simulink model "AK109_LSQ_simpFric"  (R2025a)
settings: Solver=FixedStepAuto  StartTime=0.0  StopTime=10.0  FixedStep=0.00025  RelTol=1e-3
values from neighbouring files (symbols this model uses):
  b = 1.49    [LSQ_motor_model.m]
  J = 1.59    [LSQ_motor_model.m]
  Kd = Tests(5, index)    [LSQ_motor_model.m]
  Kp = Tests(4, index)    [LSQ_motor_model.m]
  qStepSize = Tests(1, index)    [LSQ_motor_model.m]
  StepTime = 5    [LSQ_motor_model.m]
  wStart = Tests(2, index)    [LSQ_motor_model.m]
  wStepSize = Tests(3, index)    [LSQ_motor_model.m]
undefined symbols (not defined in the file or in its folder): X, Y, Z
libraries: sm_lib x7, nesl_utility x5, fl_lib x4, BalekaSSCs_lib x1
settings Model: Creator=Blue Fifth  LastModifiedBy=Gavin
settings RTWCC: GPUComputeCapability=3.5
settings ExplorerConfigSet: SimMechanicsOpenEditorOnUpdate=off

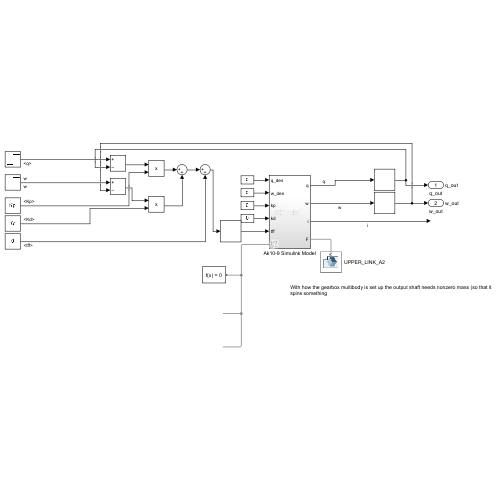
[thumbnail: Simulink's stored preview of the top-level diagram]
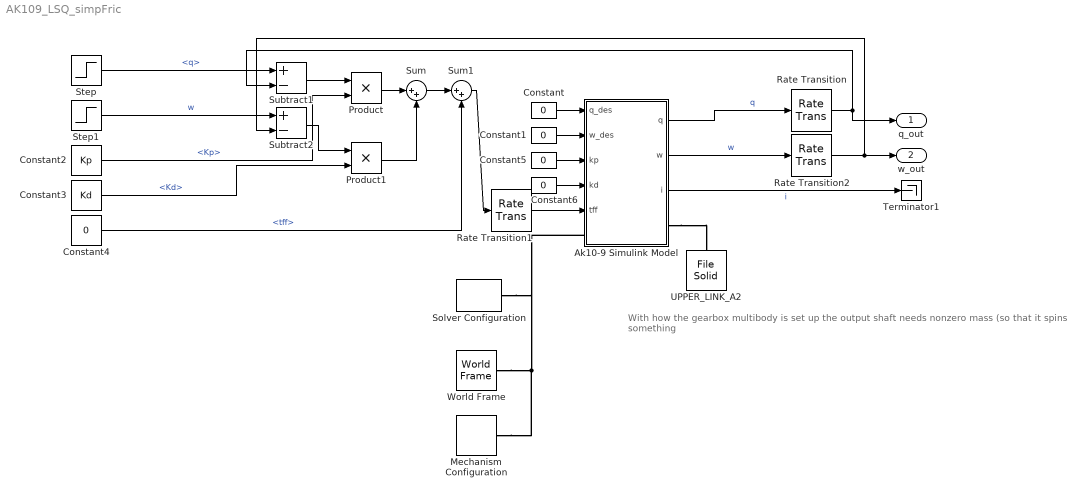
== system AK109_LSQ_simpFric ==
  note: With how the gearbox multibody is set up the output shaft needs nonzero mass (so that it spins something
  Ak10-9 Simulink Model : Subsystem  AncestorBlock=aru_toolbox/Baleka 2.5/Ak10-9 Simulink Model
  Constant{,1,4..6} (5 alike) : Constant  Value=0
  Constant2 : Constant  Value=Kp
  Constant3 : Constant  Value=Kd
  Mechanism Configuration : sm_lib/Utilities/Mechanism Configuration  UniformGravity=Constant  GravityVector=[0 0 -9.80665]  GravityVectorUnits=m/s^2  LinearizationDelta=0.001  JointModeTransitionNonlinearIterations=2
  Product : Product
  Product1 : Product
  Rate Transition : RateTransition  OutPortSampleTime=1/1000
  Rate Transition1 : RateTransition  OutPortSampleTime=1/1000
  Rate Transition2 : RateTransition  OutPortSampleTime=1/1000
  Solver Configuration : nesl_utility/Solver Configuration  PhysicalDomain=network_engine_domain  SubClassName=solver  LeftPortType=input  RightPortType=generic  Tones=[]  Harmonics=[]  SimulateNoise=off  Profile=off  UseLocalSampling=off  EnableSwitchedLinearOptims=on  FrequencyDomain=off  UseCCode=off  RelTol=0.001  AbsTol=0.001  MinStep=1e-09  ToWorkspace=off  RevertToSquareIcSolve=off  NumHomotopyIterations=100  PhasorMode=off  PhasorModeNumHarmonics=1  ConsistencySolver=NEWTON_XTOL_AFTER_FTOL  IndexReductionMethod=DerivativeReplacement  DoDC=off  ResidualTolerance=1e-09  ConsistencyTolSource=GLOBAL  ConsistencyAbsTol=0.001  ConsistencyRelTol=0.001  ConsistencyTolFactor=0.001  UseLocalSolver=off  LocalSolverChoice=NE_BACKWARD_EULER_ADVANCER  ResolveIndetEquations=on  FunctionEvalNumThread=1  LocalSolverSampleTime=0.001  DoFixedCost=off  MaxNonlinIter=3  MaxModeIter=2  ComputeImpulses=off  ImpulseIterations=2  LinearAlgebra=auto  LinearAlgebraNumThread=0  EquationFormulation=NE_TIME_EF  DelaysMemoryBudget=1024  AutomaticFiltering=on  FilteringTimeConstant=0.001  PartitionStorageMethod=AS_NEEDED  PartitionMemoryBudget=1024  PartitionMethod=ROBUST  MultibodyUseLocalSolver=off  MultibodyLocalSolverChoice=ODE1  MultibodyLocalSolverSampleTime=0.001
  Step : Step  Time=StepTime  After=qStepSize  SampleTime=0
  Step1 : Step  Time=StepTime  Before=wStart  After=wStepSize+wStart  SampleTime=0
  Subtract1 : Sum  Inputs=+-
  Subtract2 : Sum  Inputs=+-
  Sum : Sum  Inputs=|++
  Sum1 : Sum  Inputs=|++
  Terminator1 : Terminator
  UPPER_LINK_A2 : sm_lib/Body Elements/File Solid  ExtGeomFileName=leg1.STL  UnitType=Custom  ExtGeomFileUnits=mm  StepReaderType=HEX  ExportConvexHullGeometry=off  InertiaType=Custom  BasedOnType=DensityFromFile  Density=1000  DensityUnits=kg/m^3  Mass=0.001  MassUnits=g  CenterOfMass=[0 0.001 0.001]  CenterOfMassUnits=mm  MomentsOfInertia=[0 0 0]  MomentsOfInertiaUnits=g*mm^2  ProductsOfInertia=[0 0 0]  ProductsOfInertiaUnits=g*mm^2  GraphicType=FromGeometry  MarkerShape=Sphere  MarkerSize=10  GraphicVisPropType=SimpleVisualProperties  GraphicDiffuseColor=[0.6 1.0 0.6]  GraphicOpacity=1.0  GraphicSpecularColor=[0.5 0.5 0.5 1.0]  GraphicAmbientColor=[0.15 0.15 0.15 1.0]  GraphicEmissiveColor=[0.0 0.0 0.0 1.0]  GraphicShininess=75  DoExposeReferenceFrame=on  SerializedFrames=<Frames/>
  World Frame : sm_lib/Frames and Transforms/World Frame
  q_out : Outport  SignalName=q_out
  w_out : Outport  Port=2  SignalName=w_out
  wires:
  Ak10-9 Simulink Model/1(q) -> Rate Transition/1  "q"
  Ak10-9 Simulink Model/2(w) -> Rate Transition2/1  "w"
  Ak10-9 Simulink Model/3(i) -> Terminator1/1  "i"
  Rate Transition/1 -> q_out/1, Subtract1/2
  Constant/1 -> Ak10-9 Simulink Model/1(q_des)
  Constant2/1 -> Product/2  "<Kp>"
  Step/1 -> Subtract1/1  "<q>"
  Subtract2/1 -> Product1/1
  Product/1 -> Sum/1
  Subtract1/1 -> Product/1
  Sum1/1 -> Rate Transition1/1
  Product1/1 -> Sum/2
  Constant6/1 -> Ak10-9 Simulink Model/4(kd)
  Sum/1 -> Sum1/1
  Constant5/1 -> Ak10-9 Simulink Model/3(kp)
  Constant4/1 -> Sum1/2  "<tff>"
  Constant3/1 -> Product1/2  "<Kd>"
  Constant1/1 -> Ak10-9 Simulink Model/2(w_des)
  Step1/1 -> Subtract2/1  "w"
  Rate Transition1/1 -> Ak10-9 Simulink Model/5(tff)
  Rate Transition2/1 -> w_out/1, Subtract2/2
  connections:
  Ak10-9 Simulink Model/RConn1 -- UPPER_LINK_A2/RConn1
  World Frame/RConn1 -- Mechanism Configuration/RConn1 -- Ak10-9 Simulink Model/LConn1 -- Solver Configuration/RConn1

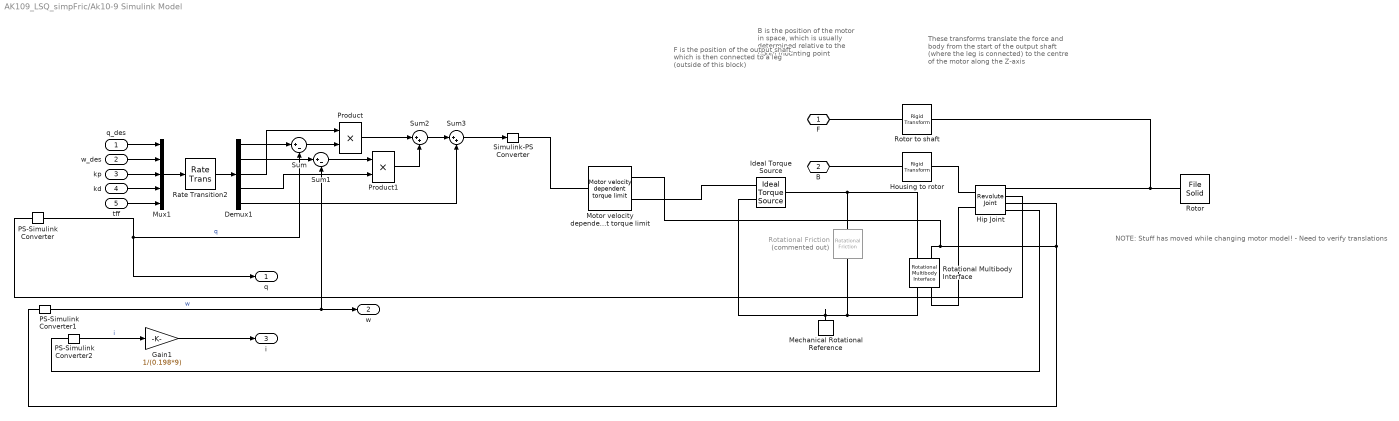
== system AK109_LSQ_simpFric/Ak10-9 Simulink Model ==
  note: These transforms translate the force and body from the start of the output shaft (where the leg is connected) to the centre of the motor along the Z-axis
  note: B is the position of the motor in space, which is usually determined relative to the boom mounting point
  note: F is the position of the output shaft, which is then connected to a leg (outside of this block)
  note: NOTE: Stuff has moved while changing motor model! - Need to verify translations
  q_des : Inport
  w_des : Inport  Port=2
  kp : Inport  Port=3
  kd : Inport  Port=4
  tff : Inport  Port=5
  Demux1 : Demux  Outputs=5
  Gain1 : Gain  Gain=1/(0.198*9)
  Hip Joint : sm_lib/Joints/Revolute Joint  JointMode=Normal  CompositeWrenchDir=BaseOnFollower  CompositeWrenchFrame=BaseFrame  SenseConstraintForce=off  SenseConstraintTorque=off  SenseTotalForce=off  SenseTotalTorque=off  PositionTargetSpecify=on  PositionTargetPriority=High  PositionTargetValue=0  PositionTargetValueUnits=rad  VelocityTargetSpecify=on  VelocityTargetPriority=High  VelocityTargetValue=0  VelocityTargetValueUnits=rad/s  EquilibriumPosition=0  EquilibriumPositionUnits=deg  SpringStiffness=0  SpringStiffnessUnits=N*m/deg  DampingCoefficient=b/10  DampingCoefficientUnits=N*m*s/rad  LowerLimitSpecify=off  LowerLimitBound=-90  LowerLimitBoundUnits=deg  LowerLimitStiffness=1e4  LowerLimitStiffnessUnits=N*m/deg  LowerLimitDamping=10  LowerLimitDampingUnits=N*m/(deg/s)  LowerLimitTransitionRegionWidth=0.1  LowerLimitTransitionRegionWidthUnits=deg  UpperLimitSpecify=off  UpperLimitBound=90  UpperLimitBoundUnits=deg  UpperLimitStiffness=1e4  UpperLimitStiffnessUnits=N*m/deg  UpperLimitDamping=10  UpperLimitDampingUnits=N*m/(deg/s)  UpperLimitTransitionRegionWidth=0.1  UpperLimitTransitionRegionWidthUnits=deg  TorqueActuationMode=InputTorque  MotionActuationMode=ComputedMotion  SensePosition=on  SenseVelocity=on  SenseAcceleration=off  SenseTorqueForce=on  SenseLowerLimitTorqueForce=off  SenseUpperLimitTorqueForce=off
  Housing to rotor : sm_lib/Frames and Transforms/Rigid Transform  RotationMethod=None  FollAlignAxisA=+X  BaseAlignAxisA=+Y  FollAlignAxisB=+Y  BaseAlignAxisB=+Z  RotationStandardAxis=+Z  RotationAngle=0.0  RotationAngleUnits=deg  RotationArbitraryAxis=[0 0 1]  RotationSequenceAxes=FollowerAxes  RotationSequence=XYX  RotationSequenceAngles=[0 0 0]  RotationSequenceAnglesUnits=deg  RotationMatrix=[1 0 0; 0 1 0; 0 0 1]  Quaternion=[1 0 0 0]  TranslationMethod=Cartesian  TranslationCartesianOffset=[0 0 -15]  TranslationCartesianOffsetUnits=mm  TranslationStandardAxis=+Z  TranslationStandardOffset=0  TranslationStandardOffsetUnits=mm  TranslationROffset=0  TranslationROffsetUnits=m  TranslationThetaOffset=0  TranslationThetaOffsetUnits=deg  TranslationZOffset=0  TranslationZOffsetUnits=m
  Ideal Torque Source : fl_lib/Mechanical/Mechanical Sources/Ideal Torque Source
  Mechanical Rotational Reference : fl_lib/Mechanical/Rotational Elements/Mechanical Rotational Reference
  Motor velocity dependent torque limit : BalekaSSCs_lib/Motor velocity dependent torque limit  t_max=54 N*m  t_rated=18 N*m  w_max=27.92 rad/s  w_rated=23.24 rad/s
      settings: InternalSimscapePortConfiguration="{\"Bottom\":[],\"Left\":[{\"id\":\"t_in\",\"label\":\"t\",\"type\":\"input\"}],\"Right\":[{\"id\":\"w\",\"label\":\"w\",\"type\":\"input\"},{\"id\":\"t_out\",\"label\":\"t\",\"type\":\"output\"}],\"Top\":[]}"
  Mux1 : Mux  Inputs=5
  PS-Simulink Converter : nesl_utility/PS-Simulink Converter  PhysicalDomain=network_engine_domain  SubClassName=ps_output  LeftPortType=input  RightPortType=output  PseudoPeriodic=off  Frequencies=[]  VectorFormat=inherit  Unit=rad  AffineConversion=off
  PS-Simulink Converter1 : nesl_utility/PS-Simulink Converter  PhysicalDomain=network_engine_domain  SubClassName=ps_output  LeftPortType=input  RightPortType=output  PseudoPeriodic=off  Frequencies=[]  VectorFormat=inherit  Unit=rad/s  AffineConversion=off
  PS-Simulink Converter2 : nesl_utility/PS-Simulink Converter  PhysicalDomain=network_engine_domain  SubClassName=ps_output  LeftPortType=input  RightPortType=output  PseudoPeriodic=off  Frequencies=[]  VectorFormat=inherit  Unit=N*m  AffineConversion=off
  Product : Product
  Product1 : Product
  Rate Transition2 : RateTransition  OutPortSampleTime=1/1000
  Rotational Friction : fl_lib/Mechanical/Rotational Elements/Rotational Friction  Commented=on  brkwy_trq=Bt N*m  brkwy_vel=0.01 rad/s  Col_trq=Ct N*m  visc_coef=b/10 N*m*s/rad  w_specify=off  w_priority=Low  w=0 rad/s  w_nominal_specify=off  w_nominal_value=1  w_nominal_unit=rad/s  t_specify=off  t_priority=Low  t=0 N*m  t_nominal_specify=off  t_nominal_value=1  t_nominal_unit=N*m
  Rotational Multibody Interface : fl_lib/Mechanical/Multibody Interfaces/Rotational Multibody Interface
  Rotor : sm_lib/Body Elements/File Solid  ExtGeomFileName=simulink-toolbox/Baleka/Meshes/AK90_10_rotor.stl  UnitType=Custom  ExtGeomFileUnits=mm  StepReaderType=HEX  ExportConvexHullGeometry=off  InertiaType=Custom  BasedOnType=Mass  Density=1  DensityUnits=kg/m^3  Mass=0  MassUnits=g  CenterOfMass=[0 0 0]  CenterOfMassUnits=mm  MomentsOfInertia=[0 0 J*1e-2]  MomentsOfInertiaUnits=kg*m^2  ProductsOfInertia=[0 0 0]  ProductsOfInertiaUnits=g*mm^2  GraphicType=FromGeometry  MarkerShape=Sphere  MarkerSize=10  GraphicVisPropType=AdvancedVisualProperties  GraphicDiffuseColor=[0.0 0.0 1.0 1.0]  GraphicOpacity=1.0  GraphicSpecularColor=[0.5 0.5 0.5 1.0]  GraphicAmbientColor=[0.15 0.15 0.15 1.0]  GraphicEmissiveColor=[0.0 0.0 0.0 1.0]  GraphicShininess=75  DoExposeReferenceFrame=on  SerializedFrames=<Frames/>
  Rotor to shaft : sm_lib/Frames and Transforms/Rigid Transform  RotationMethod=None  FollAlignAxisA=+X  BaseAlignAxisA=+Y  FollAlignAxisB=+Y  BaseAlignAxisB=+Z  RotationStandardAxis=+Z  RotationAngle=0.0  RotationAngleUnits=deg  RotationArbitraryAxis=[0 0 1]  RotationSequenceAxes=FollowerAxes  RotationSequence=XYX  RotationSequenceAngles=[0 0 0]  RotationSequenceAnglesUnits=deg  RotationMatrix=[1 0 0; 0 1 0; 0 0 1]  Quaternion=[1 0 0 0]  TranslationMethod=Cartesian  TranslationCartesianOffset=[0 0 -15]  TranslationCartesianOffsetUnits=mm  TranslationStandardAxis=+Z  TranslationStandardOffset=0  TranslationStandardOffsetUnits=mm  TranslationROffset=0  TranslationROffsetUnits=m  TranslationThetaOffset=0  TranslationThetaOffsetUnits=deg  TranslationZOffset=0  TranslationZOffsetUnits=m
  Simulink-PS Converter : nesl_utility/Simulink-PS Converter  PhysicalDomain=network_engine_domain  SubClassName=ps_input  LeftPortType=input  RightPortType=output  PseudoPeriodic=off  Frequencies=[]  NoiseDistribution=none  NoiseParameters=[]  Unit=1  AffineConversion=off  FilteringAndDerivatives=provide  SimscapeFilterOrder=1  InputFilterTimeConstant=0.001  UdotUserProvided=0
  Sum : Sum  Inputs=|+-
  Sum1 : Sum  Inputs=|+-
  Sum2 : Sum  Inputs=|++
  Sum3 : Sum  Inputs=|++
  F : PMIOPort  Side=Right
  B : PMIOPort  Port=2  Side=Left
  q : Outport
  w : Outport  Port=2
  i : Outport  Port=3
  wires:
  Gain1/1 -> i/1
  Sum3/1 -> Simulink-PS Converter/1
  Demux1/5 -> Sum3/2
  Sum2/1 -> Sum3/1
  Demux1/4 -> Product1/2
  Sum1/1 -> Product1/1
  Product1/1 -> Sum2/2
  Sum/1 -> Product/2
  Demux1/3 -> Product/1
  Product/1 -> Sum2/1
  Demux1/2 -> Sum1/1
  Demux1/1 -> Sum/1
  q_des/1 -> Mux1/1
  w_des/1 -> Mux1/2
  kp/1 -> Mux1/3
  kd/1 -> Mux1/4
  tff/1 -> Mux1/5
  Mux1/1 -> Rate Transition2/1
  Rate Transition2/1 -> Demux1/1
  PS-Simulink Converter2/1 -> Gain1/1  "i"
  PS-Simulink Converter/1 -> q/1, Sum/2  "q"
  PS-Simulink Converter1/1 -> w/1, Sum1/2  "w"
  connections:
  Hip Joint/RConn4 -- PS-Simulink Converter2/LConn1
  Rotational Multibody Interface/LConn1 -- Hip Joint/LConn2
  Motor velocity dependent torque limit/RConn2 -- Ideal Torque Source/RConn1
  Motor velocity dependent torque limit/LConn1 -- Simulink-PS Converter/RConn1
  Ideal Torque Source/LConn1 -- Rotational Multibody Interface/RConn2 -- Rotational Friction/LConn1
  Mechanical Rotational Reference/LConn1 -- Ideal Torque Source/RConn2 -- Rotational Multibody Interface/LConn2 -- Rotational Friction/RConn1
  Rotational Multibody Interface/RConn1 -- Motor velocity dependent torque limit/RConn1 -- Hip Joint/RConn3 -- PS-Simulink Converter1/LConn1
  Rotor/RConn1 -- Hip Joint/RConn1 -- Rotor to shaft/RConn1
  Hip Joint/LConn1 -- Housing to rotor/RConn1
  B/RConn1 -- Housing to rotor/LConn1
  Hip Joint/RConn2 -- PS-Simulink Converter/LConn1
  F/RConn1 -- Rotor to shaft/LConn1
